simulink subsystem "LW_noaileron_dynamic"  (R2024b)
settings: Solver=VariableStepAuto  StartTime=0.0  StopTime=10.0  RelTol=1e-3
undefined symbols (not defined in the file or in its folder): decyear, DiscIntNeverNeededParam, Earth, F, Light, LW_ANGLE, MIL, ModelFailWind_ConstWindX, ModelFailWind_ConstWindY, ModelFailWind_ConstWindZ, ModelFailWind_GustWindFreq, ModelFailWind_GustWindStrength, ModelFailWind_isConstWind, ModelFailWind_isEnable, ModelFailWind_isGustWind, ModelFailWind_isSheerWind, ModelFailWind_isTurbWind, ModelInit_AngEuler, ModelInit_PosE, ModelInit_Rads, ModelInit_RateB, ModelInit_servoRads, ModelInit_VelB, ModelParam_DeltaRatemax, ModelParam_efficiency, ModelParam_envAltitude, ModelParam_LBb, ModelParam_LBc, ModelParam_LBClp, ModelParam_LBCmq, ModelParam_LBCnr, ModelParam_LBRho, ModelParam_LBS, ModelParam_lDeltamax, ModelParam_lDeltamin, ModelParam_motorp1, ModelParam_motorp2, ModelParam_motorp3, ModelParam_motorT, ModelParam_motorUp1, ModelParam_motorUp2, ModelParam_motorUp3, ModelParam_noiseFBa, ModelParam_noiseFBaSeed, ModelParam_noiseFNa, ModelParam_noiseFNaSeed, ModelParam_noiseMNa, ModelParam_noiseMNaSeed, ModelParam_rDeltamax, ModelParam_rDeltamin, ModelParam_servoT, ModelParam_temperature, ModelParam_uavCCm, ModelParam_uavCd, ModelParam_uavJ, ModelParam_uavMass, ModelParam_use_CoesaAtmosphereModel_density, ModelParam_use_CoesaAtmosphereModel_temperature, ModelReset_Euler, ModelReset_Pos ... (+5)
libraries: simulink x5, aerolibwind2 x3, sharedtransform x2, sharedutil x2, aerolibtransform2 x1, aerolibasang x1, aerolibatmos2 x1, aerolibconvert2 x1, aerolibgravity2 x1, shared6dof x1
(part 2 of 2)

== matlab function LW_noaileron_dynamic/Environment Models/MATLAB Function1 ==
  settings: updateMethod=DISCRETE
  data: rho input; alpha output; beta output; k input; va_b input; airspeed output; qbar output; va_l output
function [alpha, beta, airspeed, qbar, va_l] = calIncidAirspeed(rho, k, va_b)
Rm = [cos(k), 0, -sin(k);
    0, 1, 0;
    sin(k), 0, cos(k)];
va_l = Rm * va_b;


airspeed = norm(va_l, 2);
sigma = 0.3;
alpha = atan2(va_l(3), va_l(1))*tanh(airspeed/sigma);
beta = asin(va_l(2) / (airspeed+sigma))*tanh(airspeed/sigma);

qbar = 0.5 * rho * airspeed ^ 2;

== matlab function LW_noaileron_dynamic/Motor and Servo Model/Subsystem/MATLAB Function ==
  settings: updateMethod=DISCRETE
  data: Ad input; Aa output; dt input; rate_max input
function Aa = servo_dynamic(Ad, dt, rate_max)
persistent Ad_last;
if isempty(Ad_last)
    Ad_last = 0;
end

Ad_rate_ref = (Ad - Ad_last) / dt;
Aa = Ad;
if Ad_rate_ref > rate_max
    Aa = Ad_last + rate_max * dt;
elseif Ad_rate_ref < -rate_max
    Aa = Ad_last - rate_max * dt;
end

Ad_last = Aa;
end

== matlab function LW_noaileron_dynamic/Motor and Servo Model/Subsystem1/MATLAB Function ==
  settings: updateMethod=DISCRETE
  data: Ad input; Aa output; dt input; rate_max input
function Aa = servo_dynamic(Ad, dt, rate_max)
persistent Ad_last;
if isempty(Ad_last)
    Ad_last = 0;
end

Ad_rate_ref = (Ad - Ad_last) / dt;
Aa = Ad;
if Ad_rate_ref > rate_max
    Aa = Ad_last + rate_max * dt;
elseif Ad_rate_ref < -rate_max
    Aa = Ad_last - rate_max * dt;
end

Ad_last = Aa;
end

== matlab function LW_noaileron_dynamic/Environment Models/Wind Models/GustWindModel ==
  settings: updateMethod=DISCRETE
  data: t input; gWind output; isGustWind input; GustWindStrength input; GustWindFreq input; turb input
function gWind = GustWindModel(t,isGustWind,GustWindStrength,GustWindFreq,turb)

if(GustWindFreq<1)
    GustWindFreq=1;
end
timeVel=60/GustWindFreq;

vmax=GustWindStrength;

persistent t0;
if isempty(t0)
    t0=0;
end

persistent isInGust;
if isempty(isInGust)
    isInGust=0;
end

persistent t1;
if isempty(t1)
    t1=2;
end

persistent a;
if isempty(a)
    a=0.5;
end

persistent ang;
if isempty(ang)
    ang=0;
end

persistent wlast;
if isempty(wlast)
    wlast=vmax*0.5;
end

persistent wNow;
if isempty(wNow)
    wNow=1.4*0.8*vmax;
end


if isGustWind&&isInGust<0.5
    t0=t;
    t1=timeVel*(3/4+1/2*rand(1));
    a=1/4+1/2*rand(1);
    ang=pi*2*rand(1);
    wlast=wNow;
    wNow=1.2*(rand(1)*0.5+0.5)*vmax;
    
    isInGust=1;
end

if ~isGustWind
    isInGust=0;
end

gWind=[0;0;0];

if(t<t0+t1*a)
    gWindMag=(wNow-wlast)/2*(1-cos((t-t0)/(t1*a)*pi))+wlast;
else
    gWindMag=wNow;
end

if abs(t-(t0+t1))<0.05
    rng(t*1000);
    t0=t;
    t1=timeVel*(3/4+1/2*rand(1));
    a=1/4+1/2*rand(1);
    ang=ang+0.1*pi*rand(1);
    wlast=wNow;
    wNow=1.2*(rand(1)*0.5+0.5)*vmax;
end

gWind(1)=gWindMag*cos(ang)*0.8+turb(1)*0.4;
gWind(2)=gWindMag*sin(ang)*0.8+turb(2)*0.4;
gWind(3)=turb(3)*0.4;

== matlab function LW_noaileron_dynamic/Forces and Moments/Aerodynamics and torque ==
  data: alpha input size=1; qbar input; va_l input; wb input size=[3,1]; vb input size=[3,1]; C_D input size=1; C_Y input size=1; C_L input size=1; C_l input size=1; C_m input size=1; C_n input size=1; USE_AeroCoefficient parameter size=1; Fa output size=[3,1]; Ma output size=[3,1]; ModelParam_LBClp parameter size=1; ModelParam_LBCmq parameter size=1; ModelParam_LBCnr parameter size=1; Fa_l output size=[3,1]; Ma_l output size=[3,1]; ModelParam_LBS parameter size=1; ModelParam_LBc parameter size=1; ModelParam_LBb parameter size=1; LW_ANGLE parameter size=1; ModelParam_uavCd parameter size=[3,1]; ModelParam_uavCCm parameter size=[3,1]; ModelParam_LBRho parameter
function [Fa,  Ma, Fa_l, Ma_l] = fcn(alpha, qbar,va_l, wb, vb, C_D, C_Y, C_L, C_l, C_m, C_n, USE_AeroCoefficient,...
    ModelParam_LBClp, ModelParam_LBCmq, ModelParam_LBCnr, ModelParam_LBS, ModelParam_LBc, ModelParam_LBb, LW_ANGLE, ModelParam_uavCd, ModelParam_uavCCm, ModelParam_LBRho)
%Function description;
% S: 机翼的俯视面积
% c: 机翼的平均弦长
% b: 翼展
% C_L, C_D, C_m, C_Y, C_l, C_n: 空气动力学系数
% qbar: 0.5*rho*Va^2 ,rho: 空气密度 Va: 空速
% incid: 迎角，侧滑角
% kappa: 安装角

%纵向
if ~USE_AeroCoefficient
    qbar = 0;
end

S = ModelParam_LBS;
c = ModelParam_LBc;
b = ModelParam_LBb;
rho = ModelParam_LBRho;
kappa  = LW_ANGLE*pi/180;
C_d = ModelParam_uavCd;
C_md = ModelParam_uavCCm;

F_lift = qbar*S*C_L;
F_drag = qbar*S*C_D;
m = qbar*S*c*C_m;
%将力从气动坐标系转换到机体坐标系
lambda = alpha - kappa;
f_x = cos(lambda)*(-F_drag) - sin(lambda)*(-F_lift);
f_z = sin(lambda)*(-F_drag) + cos(lambda)*(- F_lift);
%横向
f_y = qbar*S*C_Y;
l_s = qbar*S*b*C_l;
n_s = qbar*S*b*C_n;
l = cos(kappa)*l_s + sin(kappa)*n_s;
n = -sin(kappa)*l_s + cos(kappa)*n_s;


%φ-theory
u = 1;
Cd0 = 0.26;
Cy0 = 0.0;
delta_r = 0;
Comega = [b 0 0; 0 c 0; 0 0 b];

R_lb = [cos(kappa), 0 , -sin(kappa);
    0,     1 ,    0;
    sin(kappa), 0 ,  cos(kappa)];
wl = R_lb*wb;
vl = R_lb*vb;
Va_norm = sqrt(va_l'*va_l);
eta = sqrt(Va_norm^2 + u*c*(wl'*wl));
AR = b^2/S;
phi_fv = [Cd0 0 0; 0 Cy0 0 ; 0 0 0.5*pi*AR/(1+sqrt(1+(AR/2)^2))+Cd0];
phi_fw = [0 0 0;0 0 1/b*delta_r*Cy0;0 -1/c*delta_r*(pi*AR/(1+sqrt(1+(AR/2)^2)) + Cd0) 0];
phi_mv = [0 0 0; 0 0 -1/c*delta_r*(pi*AR/(1+sqrt(1+(AR/2)^2)) + Cd0);0 1/b*delta_r*Cy0 0];
phi_mw = 0.5*[ModelParam_LBClp 0 0; 0 ModelParam_LBCmq 0;0 0 ModelParam_LBCnr];
Fa_l = -0.5*rho*S*eta*(phi_fv*vl + phi_fw*Comega*wl);
Ma_l = -0.5*rho*S*eta*(Comega*phi_mv*vl + Comega*phi_mw*Comega*wl);

if ~USE_AeroCoefficient
    %不使用固定翼中气动系数，而是使用简单的阻力和阻力矩系数
    Fa= -C_d .* va_l.*abs(va_l);
    
    % 计算空气产生的力矩
    Ma = -C_md.* wb.*abs(wb);
else
    Fa = [f_x, f_y, f_z]';
    Ma = [l, m, n]' - R_lb'*Ma_l;
end


end

== matlab function LW_noaileron_dynamic/Forces and Moments/MATLAB Function ==
  settings: updateMethod=DISCRETE
  data: Wb input; DCM input; Xe input; Ve input; Quet input; euler input; terrainZ input; landed input; mg input; F_env output size=[3,1]; M_env output size=[3,1]; ModelInit_AngEuler parameter
function [F_env, M_env] = fcn( Wb,DCM, Xe, Ve, Quet, euler, terrainZ, landed, mg, ModelInit_AngEuler)
persistent hold_yaw_flag land_yaw
if isempty(land_yaw) || isempty(hold_yaw_flag)
    land_yaw = ModelInit_AngEuler(3);
    hold_yaw_flag = true;
end
if landed && ~hold_yaw_flag
    land_yaw = euler(3);
    hold_yaw_flag = true;
end

%计算地面产生的力和力矩
z = Xe(3) - terrainZ;
F_ground=[0;0;0];
M_ground=[0;0;0];
if landed
    if z < 0.01
         F_ground(3) = -mg(3)- 1*z- 10*Ve(3); 
    elseif z<0.04
        F_ground(3)=-mg(3)-0.5*z-20*Ve(3); 
    else
         F_ground(3)=-mg(3)-1.0*z-50*Ve(3); 
    end

    F_ground(1)=-1000*Ve(1);
    F_ground(2)=-1000*Ve(2);
    F_ground = F_ground(:);
    M_ground=-200*[Quet(2);Quet(3);Quet(4)]-10*Wb;
    %M_ground=-1*[euler(1);euler(2); (euler(3)-land_yaw)]-2*Wb;
else
    hold_yaw_flag = false;
end     

F_env = DCM'*(mg + F_ground);
M_env = M_ground;

== matlab function LW_noaileron_dynamic/Forces and Moments/Propeller Model ==
  data: w input; Va input; Fp output size=[3,1]; Mp output size=[3,1]; wb input; USE_PROPELLER_MODEL1 parameter; Ga output size=[3,1]; ModelParam_propellerkT0 parameter; ModelParam_propellerkTvarpi parameter; ModelParam_propellerkTV parameter; ModelParam_propellerkTvarpi2 parameter; ModelParam_propellerkTvarpiV parameter; ModelParam_propellerkTV2 parameter; ModelParam_propellerkM0 parameter; ModelParam_propellerkMvarpi parameter; ModelParam_propellerkMV parameter; ModelParam_propellerkMvarpi2 parameter; ModelParam_propellerkMvarpiV parameter; ModelParam_propellerkMV2 parameter; ModelParam_rotorCm parameter; ModelParam_rotorCt parameter; ModelParam_rotordx parameter; ModelParam_rotordy parameter; ModelParam_rotorEta parameter; ModelParam_motorJm parameter
function [Fp, Mp, Ga] = fcn(w, Va, wb, USE_PROPELLER_MODEL1 ,ModelParam_propellerkT0, ModelParam_propellerkTvarpi, ModelParam_propellerkTV, ...
    ModelParam_propellerkTvarpi2, ModelParam_propellerkTvarpiV, ModelParam_propellerkTV2, ...
    ModelParam_propellerkM0, ModelParam_propellerkMvarpi, ModelParam_propellerkMV, ...
    ModelParam_propellerkMvarpi2, ModelParam_propellerkMvarpiV, ModelParam_propellerkMV2, ...
    ModelParam_rotorCm, ModelParam_rotorCt, ModelParam_rotordx, ModelParam_rotordy, ModelParam_rotorEta, ModelParam_motorJm)...
    %Function description;
%  According to the rotational speed, the force and torque provided by the propeller
%  to the quadrotor-X aircraft are calculated. The distribution of the quadrotor motor is as follows:
%3↓   1↑
%  \ /
%  / \
%4↑   2↓
%↑ stands for counterclockwise and ↓stands for clockwise
%Input：
%  w: Motor speed，unit：rad/s
%  R: Body radius(m)
%  Cm: torque coefficient
%  Ct: thrust coefficient
%  Vb: Aircraft speed in the body coordinate system
%  Cd: Damping coefficient
%  wb: Angular velocity in the body coordinate system
%  Cdm: Damping moment coefficient vector
%  Jrp:  Moment of inertia of motor rotor + propeller
%Output:
%  Fb: thrust under the body coordinate system
%  Fd: air resistance under the body coordinate system
%  Mb: torque under the body coordinate system
%  Md: aerodynamic moment
%  Ga: gyro moment

Cm = ModelParam_rotorCm;
dx = ModelParam_rotordx;
dy = ModelParam_rotordy;
eta = ModelParam_rotorEta;
Jrp = ModelParam_motorJm;
Ct = ModelParam_rotorCt;
%Calculating gyro moment
Ga = zeros(3,1);
Ga(1) = Jrp*wb(2)*( w(1) - w(2) - w(3) + w(4));
Ga(2) = Jrp*wb(1)*(-w(1) + w(2) + w(3) - w(4));

w = w(:);

if USE_PROPELLER_MODEL1
    M_rctcm = [-dy*Ct*cos(eta),  -dy*Ct*cos(eta), dy*Ct*cos(eta), dy*Ct*cos(eta);
        dx*Ct*cos(eta), -dx*Ct*cos(eta), dx*Ct*cos(eta), -dx*Ct*cos(eta);
        Cm+dx*sin(eta), -Cm-dx*sin(eta), -Cm - dx*sin(eta), Cm+dx*sin(eta)];
    
    Mp = M_rctcm*(w.^2);  %torque
    
    Fp = [0 0 0 0;
        sin(eta) sin(eta) -sin(eta) -sin(eta);
        -cos(eta) -cos(eta) -cos(eta) -cos(eta)]*Ct*(w.^2);  %thrust
else
    w = w*3/(16*pi);
    T = ModelParam_propellerkT0*ones(4,1) + ModelParam_propellerkTvarpi*w + ModelParam_propellerkTV*Va*ones(4,1) + ...
        ModelParam_propellerkTvarpi2*w.*w + ModelParam_propellerkTvarpiV*w*Va + ModelParam_propellerkTV2*Va^2*ones(4,1);
    Fp = [0 0 0 0;
        sin(eta) sin(eta) -sin(eta) -sin(eta);
        -cos(eta) -cos(eta) -cos(eta) -cos(eta)]*T;  %thrust
    M = ModelParam_propellerkM0*ones(4,1) + ModelParam_propellerkMvarpi*w + ModelParam_propellerkMV*Va*ones(4,1) + ...
        ModelParam_propellerkMvarpi2*w.*w + ModelParam_propellerkMvarpiV*w*Va + ModelParam_propellerkMV2*Va^2*ones(4,1);
    M_rctcm = [-dy*cos(eta),  -dy*cos(eta), dy*cos(eta), dy*cos(eta);
        dx*cos(eta), -dx*cos(eta), dx*cos(eta), -dx*cos(eta);
        dx*sin(eta), -dx*sin(eta), -dx*sin(eta), dx*sin(eta)]*T;
    
    Mp = M_rctcm +[0 0 0 0;0 0 0 0;1 1 -1 -1]*M;  %torque
end
end

== matlab function LW_noaileron_dynamic/Motor and Servo Model/throttle2rads ==
  data: throttle input; y output; ModelParam_motorUp1 parameter; ModelParam_motorUp2 parameter; ModelParam_motorUp3 parameter; ModelParam_efficiency parameter; Ub input
function y = fcn(throttle,ModelParam_motorUp1, ModelParam_motorUp2, ModelParam_motorUp3, ModelParam_efficiency, Ub)

throttle = throttle*ModelParam_efficiency*Ub;

y = ModelParam_motorUp1*throttle^2 + ModelParam_motorUp2*throttle + ModelParam_motorUp3;

== matlab function LW_noaileron_dynamic/Motor and Servo Model/throttle2rads1 ==
  data: throttle input; y output; ModelParam_motorp1 parameter; ModelParam_motorp2 parameter; ModelParam_motorp3 parameter; ModelParam_efficiency parameter; aUb_ input
function y = fcn(throttle,ModelParam_motorp1, ModelParam_motorp2, ModelParam_motorp3, ModelParam_efficiency, aUb_)

throttle = throttle*ModelParam_efficiency;
y = ModelParam_motorp1*throttle^2 + ModelParam_motorp2*throttle + ModelParam_motorp3;

== matlab function LW_noaileron_dynamic/Motor and Servo Model/throttle2rads2 ==
  data: aUb_ input; throttle input; y output; ModelParam_motorp1 parameter; ModelParam_motorp2 parameter; ModelParam_motorp3 parameter; ModelParam_efficiency parameter
function y = fcn(aUb_, throttle,ModelParam_motorp1, ModelParam_motorp2, ModelParam_motorp3, ModelParam_efficiency)

throttle = throttle*ModelParam_efficiency;
y = ModelParam_motorp1*throttle^2 + ModelParam_motorp2*throttle + ModelParam_motorp3;

== matlab function LW_noaileron_dynamic/Motor and Servo Model/throttle2rads3 ==
  data: aUb_ input; throttle input; y output; ModelParam_motorp1 parameter; ModelParam_motorp2 parameter; ModelParam_motorp3 parameter; ModelParam_efficiency parameter
function y = fcn(aUb_, throttle,ModelParam_motorp1, ModelParam_motorp2, ModelParam_motorp3, ModelParam_efficiency)

throttle = throttle*ModelParam_efficiency;
y = ModelParam_motorp1*throttle^2 + ModelParam_motorp2*throttle + ModelParam_motorp3;

== matlab function LW_noaileron_dynamic/Rigid Model/WSH/6DOF (Quaternion)/Calculate the rotation matrix and Euler angle/Euler angle to quaternion ==
  data: EulerAngle input; q output
function q = fcn(EulerAngle)
%Function description:
%  Get quaternions from Euler angle
q0 =  cos(EulerAngle(1)/2)*cos(EulerAngle(2)/2)*cos(EulerAngle(3)/2) + sin(EulerAngle(1)/2)*sin((EulerAngle(2)/2))*sin((EulerAngle(3)/2));
q1 = sin(EulerAngle(1)/2)*cos(EulerAngle(2)/2)*cos(EulerAngle(3)/2) - cos(EulerAngle(1)/2)*sin((EulerAngle(2)/2))*sin((EulerAngle(3)/2));
q2 = cos(EulerAngle(1)/2)*sin(EulerAngle(2)/2)*cos(EulerAngle(3)/2) + sin(EulerAngle(1)/2)*cos((EulerAngle(2)/2))*sin((EulerAngle(3)/2));
q3 = cos(EulerAngle(1)/2)*cos(EulerAngle(2)/2)*sin(EulerAngle(3)/2) - sin(EulerAngle(1)/2)*sin((EulerAngle(2)/2))*cos((EulerAngle(3)/2));
q = [q0 q1 q2 q3]';

== matlab function LW_noaileron_dynamic/Rigid Model/WSH/6DOF (Quaternion)/Calculate the rotation matrix and Euler angle/Quaternion to Euler ==
  data: q input; euler output
function euler = fcn(q)
 %Function description;
%  Quaternion to Euler
phi = atan2(2*(q(1)*q(2) + q(3)*q(4)), (1 - 2*(q(2)*q(2) + q(3)*q(3))));
theta = asin(max(min(2*(q(1)*q(3) - q(2)*q(4)),1),-1));
psi = atan2(2*(q(1)*q(4) + q(2)*q(3)), (1 - 2*(q(3)*q(3) + q(4)*q(4))));
euler = [phi theta psi]';

== matlab function LW_noaileron_dynamic/Rigid Model/WSH/6DOF (Quaternion)/Calculate the rotation matrix and Euler angle/Quaternion to rotation matrix ==
  data: q input; Reb output
function Reb = fcn(q)
%Function description;
%  The rotation matrix of the body coordinate system to the geodetic coordinate system is obtained from the quaternion
Reb = [q(1)*q(1) + q(2)*q(2) - q(3)*q(3) - q(4)*q(4), 2*(q(2)*q(3) - q(1)*q(4)), 2*(q(2)*q(4) + q(1)*q(3))
       2*(q(2)*q(3) + q(1)*q(4)), q(1)*q(1) - q(2)*q(2) + q(3)*q(3) - q(4)*q(4), 2*(q(3)*q(4) - q(1)*q(2))
       2*(q(2)*q(4) - q(1)*q(3)), 2*(q(3)*q(4) + q(1)*q(2)), q(1)*q(1) - q(2)*q(2) - q(3)*q(3) + q(4)*q(4)];

== matlab function LW_noaileron_dynamic/Rigid Model/WSH/6DOF (Quaternion)/Calculate the rotation matrix and Euler angle/Quaternions model ==
  data: pqr input; qdot output; q input
function qdot = fcn(pqr, q)
%Function description;
%  Quaternions model
qdot = 0.5*[0, -pqr(1), -pqr(2), -pqr(3); pqr(1), 0, pqr(3), -pqr(2); pqr(2), -pqr(3), 0, pqr(1); pqr(3), pqr(2), -pqr(1), 0]*q;

== matlab function LW_noaileron_dynamic/Environment Models/Wind Models/MATLAB Function ==
  data: timestamp input; y output
function y = fcn(timestamp)


i = fix((timestamp - 10)/30);
y = [0 0 30*i];

== matlab function LW_noaileron_dynamic/Aerodynamic Coefficients/aerodynamic coefficients ==
  data: incid input; wb input; C_D output; delta input; LW_ANGLE parameter; ModelParam_LBb parameter; ModelParam_LBc parameter; AERO_COEFFICIENT parameter; C_Y output; C_L output; C_l output; C_m output; C_n output; ModelParam_LBCY0 parameter; ModelParam_LBCYB parameter; ModelParam_LBCl0 parameter; ModelParam_LBClB parameter; ModelParam_LBCl_d parameter; ModelParam_LBCm_d parameter; ModelParam_LBCn0 parameter; ModelParam_LBCnB parameter; ModelParam_LBCn_d parameter; ModelParam_LBCmq parameter; ModelParam_LBCnr parameter; ModelParam_LBClp parameter; ModelParam_pu_alpha0 parameter; ModelParam_pu_c1 parameter; ModelParam_pu_c0 parameter; ModelParam_pu_c2 parameter; ModelParam_pu_c3 parameter; ModelParam_pu_kL parameter; ModelParam_pu_kD parameter; ModelParam_pu_breaks parameter; ModelParam_pu_coefs parameter; ModelParam_pu_cl0 parameter; C_m0 output; C_me output
function [C_D, C_Y, C_L, C_l, C_m, C_n,C_m0, C_me] = fcn(incid, wb, delta, ...
    LW_ANGLE, ModelParam_LBb, ModelParam_LBc, AERO_COEFFICIENT, ...
    ModelParam_LBCY0, ModelParam_LBCYB, ModelParam_LBCl0, ModelParam_LBClB, ModelParam_LBCl_d, ModelParam_LBCm_d, ModelParam_LBCn0, ModelParam_LBCnB, ModelParam_LBCn_d, ModelParam_LBCmq, ModelParam_LBCnr, ModelParam_LBClp, ...
    ModelParam_pu_alpha0, ModelParam_pu_c1, ModelParam_pu_c0, ModelParam_pu_c2, ModelParam_pu_c3, ModelParam_pu_kL, ModelParam_pu_kD, ModelParam_pu_breaks, ModelParam_pu_coefs, ModelParam_pu_cl0)

    alpha = incid(1);
    beta = incid(2);
    Va = incid(3);
    
    if isnan(beta)
        beta = 0;
    end
%     maxBeta = 30 * pi / 180;
%     if beta > maxBeta
%         beta = maxBeta;
%     elseif beta < -maxBeta
%         beta = -maxBeta;
%     end
    if Va < 1
        Va = 1;
    end
    kk = LW_ANGLE*pi/180;
    Rlb = [cos(kk), 0, -sin(kk);
        0, 1, 0;
        sin(kk), 0, cos(kk)];
    delta_a = delta(2);
    delta_e = delta(1);
    wl = Rlb * wb;
    
    C_Y = ModelParam_LBCY0 + ModelParam_LBCYB * beta;
    C_l = ModelParam_LBCl0 + ModelParam_LBClB * beta + ModelParam_LBClp * ModelParam_LBb / (2 * Va) * wl(1) + ModelParam_LBCl_d * delta_a;
    C_n = ModelParam_LBCn0 + ModelParam_LBCnB * beta + ModelParam_LBCnr * ModelParam_LBb / (2 * Va) * wl(3) + ModelParam_LBCn_d * delta_a;
   
    %%% 经验公式
    alpha0 = ModelParam_pu_alpha0; %失速角度
    c0 = ModelParam_pu_c0; % 最小阻力
    c1 = ModelParam_pu_c1; %失速后最高升力，阻力
    CL0 = ModelParam_pu_cl0; % 0迎角升力
    Cla = ModelParam_pu_c2; %小迎角升力变化率
    c3 = ModelParam_pu_c3; % 小迎角阻力变化率
    kL = ModelParam_pu_kL;
    kD = ModelParam_pu_kD; %升力、阻力切换
    CL_l = c1*sin(alpha)*cos(alpha);
    CD_l = c0 + c1*sin(alpha).^2;

    CL_s = CL0+Cla.*sin(alpha)*cos(alpha);
    CD_s = c0+c3*sin(alpha).^2;
    sigmaL = (1+tanh(kL*alpha0^2-kL*alpha.^2))./(1+tanh(kL*alpha0^2));
    sigmaD = (1+tanh(kD*alpha0^2-kD*alpha.^2))./(1+tanh(kD*alpha0^2));
    
    if AERO_COEFFICIENT == int8(1) %post-stall
        C_L = CL_l;
        C_D = CD_l;
    elseif AERO_COEFFICIENT == int8(2) %pre-stall
        C_L = CL_s;
        C_D = CD_s;
    else %mix
        C_L = (1-sigmaL).*CL_l + sigmaL.*CL_s;
        C_D = (1-sigmaD).*CD_l+ sigmaD.*CD_s;
    end

    pp = mkpp(ModelParam_pu_breaks,ModelParam_pu_coefs);
    C_m = ppval(pp, alpha) + ModelParam_LBCmq * ModelParam_LBc / (2 * Va) * wl(2) + ModelParam_LBCm_d * delta_e;
    C_m0 = ppval(pp, alpha) + ModelParam_LBCmq * ModelParam_LBc / (2 * Va) * wl(2);
    C_me = ModelParam_LBCm_d * delta_e;
    %C_m = 0;
     
end
